simulink model "RLload"  (R2024a)
settings: Solver=VariableStepAuto  StartTime=0.0  StopTime=10.0  RelTol=1e-3
libraries: spsDetailedThyristorLib x4, spsCurrentMeasurementLib x2, spsVoltageMeasurementLib x2, spsACVoltageSourceLib x1, spsMeanLib x1, spsSeriesRLCBranchLib x1, sps_lib x1
settings Model: Creator=yashg  LastModifiedBy=yashg

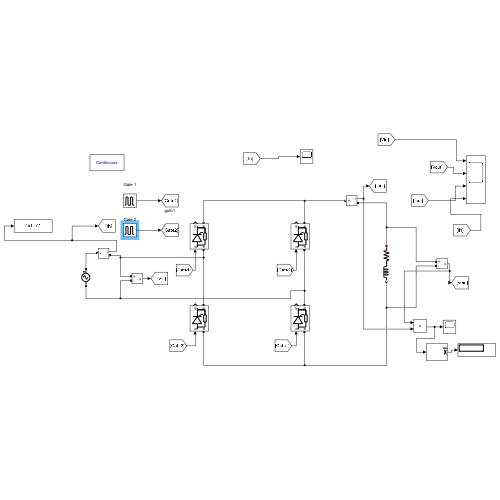
[thumbnail: Simulink's stored preview of the top-level diagram]
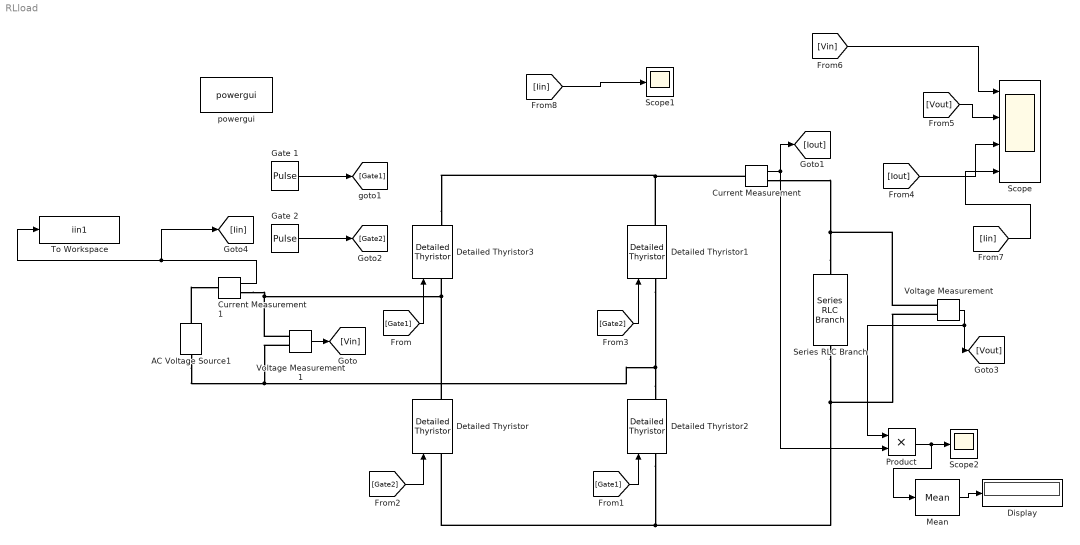
== system RLload ==
  AC Voltage Source1 : spsACVoltageSourceLib/AC Voltage Source  Amplitude=220  Phase=0  Frequency=50  SampleTime=0  Measurements=None  BusType=swing  Pref=10e3  Qref=0  Qmin=-inf  Qmax=+inf
  Current Measurement : spsCurrentMeasurementLib/Current Measurement  PhasorSimulation=off  OutputType=Complex  PSBequivalent=0
  Current Measurement1 : spsCurrentMeasurementLib/Current Measurement  PhasorSimulation=off  OutputType=Complex  PSBequivalent=0
  Detailed Thyristor{,1..3} (4 alike) : spsDetailedThyristorLib/Detailed Thyristor  Ron=0.001  Lon=1e-3  Vf=0.8  IL=0.1  Tq=100e-6  IC=0  Rs=500  Cs=250e-9  Measurements=on
      settings: LibrarySourceBlock=sps_lib/Power Electronics/Detailed Thyristor
  Display : Display
  "Gate 1 " : DiscretePulseGenerator  PulseType=Time based  Period=0.02  PulseWidth=50  PhaseDelay=0.001667
  Gate 2 : DiscretePulseGenerator  PulseType=Time based  Period=0.02  PulseWidth=50  PhaseDelay=0.011667
  Mean : spsMeanLib/Mean  Freq=60  Vinit=0  Ts=0
  Product : Product
  Scope : Scope  NumInputPorts=4
  Scope1 : Scope
  Scope2 : Scope
  Series RLC Branch : spsSeriesRLCBranchLib/Series RLC Branch  LConnTagsString=__new0  RConnTagsString=__new0  BranchType=RL  Resistance=20  Inductance=0.01  SetiL0=off  InitialCurrent=0  Capacitance=1e-6  Setx0=off  InitialVoltage=0  Measurements=None
  To Workspace : ToWorkspace  VariableName=iin1  SaveFormat=Timeseries  SampleTime=-1
  Voltage Measurement : spsVoltageMeasurementLib/Voltage Measurement  PhasorSimulation=off  OutputType=Complex  PSBequivalent=0
  Voltage Measurement1 : spsVoltageMeasurementLib/Voltage Measurement  PhasorSimulation=off  OutputType=Complex  PSBequivalent=0
  powergui : sps_lib/powergui  Priority=1  SimulationMode=Continuous  SampleTime=50e-6  frequency=60  Iterations=50  frequencyindice=50  Pbase=100e6  ErrMax=1e-4  UnitsV=kV  UnitsW=MW  buscounter=0  FunctionMessages=off  echomessages=off  EnableUseOfTLC=off  CurrentSourceSwitches=off  DisableSnubberDevices=off  DisableRonSwitches=off  DisableVfSwitches=off  DisplayEquations=off  AutomaticDiscreteSolvers=off  SolverType=Tustin/Backward Euler (TBE)  Interpol=off  ExternalGateDelay=off  methode=off  Ts=100  x0status=blocks  SPID=on  SwTol=0  HookPort=off  NonlinearTolerance=1e-4  nMaxIteration=100  ContinueOnMaxIteration=off  RestoreLinks=warning  ResistiveCurrentMeasurement=off  Frange=[0:2:500]  Ylog=off  Xlog=on  ShowGrid=off  save=off  variable=ZData  structure=0  ZoomFFT=off  StartTime=0.0  cycles=1  DisplayStyle=1  fundamental=60  FreqAxis=off  MaxFrequency=1000  frequencyindicesteady=1  RmsSteady=1  display=off
  wires:
  Product/1 -> Mean/1, Scope2/1
  Current Measurement1/1 -> To Workspace/1, [Iin]
  Mean/1 -> Display/1
  [Gate1] -> Detailed Thyristor3/1
  [Iin] -> Scope1/1
  [Gate2] -> Detailed Thyristor/1
  [Iin] -> Scope/4
  [Vout] -> Scope/2
  [Iout] -> Scope/3
  Voltage Measurement/1 -> Product/1, [Vout]
  Voltage Measurement1/1 -> [Vin]
  [Gate1] -> Detailed Thyristor2/1
  Current Measurement/1 -> [Iout], Product/2
  [Gate2] -> Detailed Thyristor1/1
  [Vin] -> Scope/1
  "Gate 1 "/1 -> [Gate1]
  Gate 2/1 -> [Gate2]
  connections:
  Series RLC Branch/RConn1 -- Detailed Thyristor2/LConn1 -- Detailed Thyristor/LConn1 -- Voltage Measurement/LConn2
  Series RLC Branch/LConn1 -- Current Measurement/RConn1 -- Voltage Measurement/LConn1
  Detailed Thyristor3/RConn1 -- Detailed Thyristor1/RConn1 -- Current Measurement/LConn1
  Detailed Thyristor/RConn1 -- Detailed Thyristor3/LConn1 -- Voltage Measurement1/LConn1 -- Current Measurement1/RConn1
  Detailed Thyristor2/RConn1 -- Detailed Thyristor1/LConn1 -- Voltage Measurement1/LConn2 -- AC Voltage Source1/LConn1
  AC Voltage Source1/RConn1 -- Current Measurement1/LConn1
